simulink model "lmod1"  (R2019a)
settings: Solver=VariableStepAuto  StartTime=0.0  StopTime=10.0  RelTol=1e-3
settings Model: Creator=83621  LastModifiedBy=83621

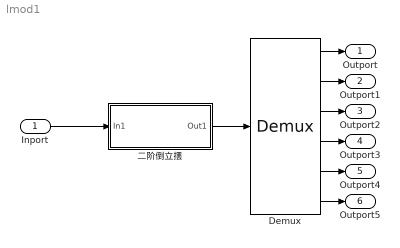
== system lmod1 ==
  Inport : Inport
  Demux : Demux  Outputs=6
  二阶倒立摆 : Subsystem  mask{m0=1.32, m1=0.132, m2=0.04, j1=0.0036, j2=0.004, l1=0.27, l2=0.09, l=0.18, f0=6.7697, f1=0.0007056, f2=0.0007056, g0=1, g=9.8}
      mask DialogControl name1 Prompt: name1
  Outport : Outport
  Outport1 : Outport  Port=2
  Outport2 : Outport  Port=3
  Outport3 : Outport  Port=4
  Outport4 : Outport  Port=5
  Outport5 : Outport  Port=6
  wires:
  Inport/1 -> 二阶倒立摆/1(In1)
  二阶倒立摆/1(Out1) -> Demux/1
  Demux/1 -> Outport/1
  Demux/2 -> Outport1/1
  Demux/3 -> Outport2/1
  Demux/4 -> Outport3/1
  Demux/5 -> Outport4/1
  Demux/6 -> Outport5/1

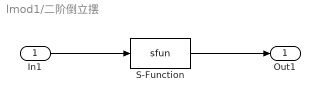
== system lmod1/二阶倒立摆 ==
  In1 : Inport
  S-Function : S-Function  FunctionName=sfun  Parameters=m0,m1,m2,j1,j2,l1,l2,l,f0,f1,f2,g0,g  SFunctionDeploymentMode=off  EnableBusSupport=off
  Out1 : Outport
  wires:
  In1/1 -> S-Function/1
  S-Function/1 -> Out1/1
